simulink subsystem "HeaterDummy"  (R2024b)
settings: Solver=VariableStepAuto  StartTime=0.0  StopTime=10.0  RelTol=1e-3
undefined symbols (not defined in the file or in its folder): batteryHeater
libraries: fl_lib x3, nesl_utility x1
Description:
  | Minimal heater stub with fixed electrical load. Draws constant current (P_max/V_nom) when heater is active (cmdHeater=1). Coolant passes through with no heat exchange. Same port interface as Heater.slx.
settings Model: Creator=jjha  LastModifiedBy=jjha

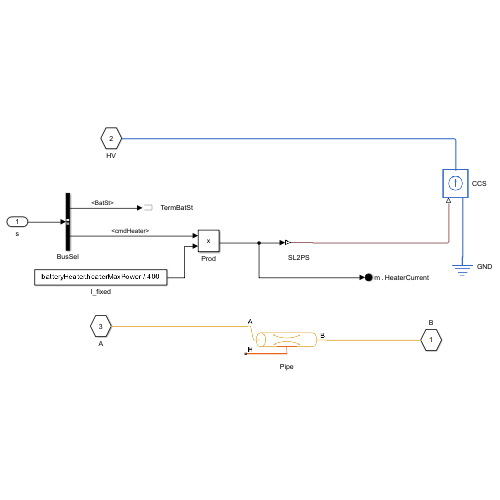
[thumbnail: Simulink's stored preview of the top-level diagram]
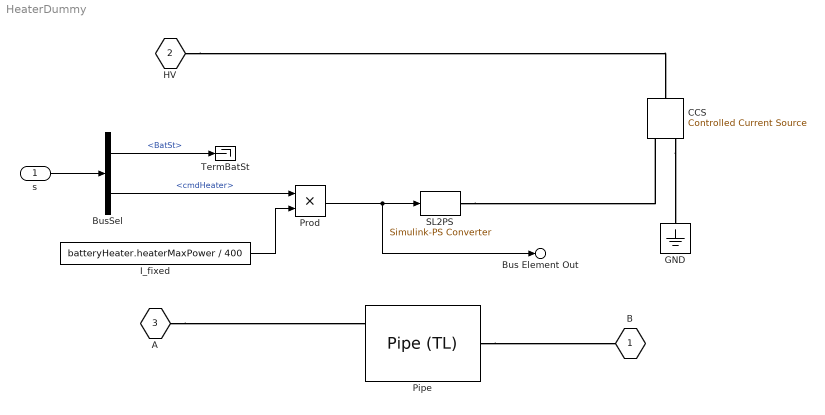
== system HeaterDummy ==
  s : Inport
  BusSel : BusSelector  OutputSignals=BatSt,cmdHeater
  CCS : fl_lib/Electrical/Electrical Sources/Controlled Current Source
  GND : fl_lib/Electrical/Electrical Elements/Electrical Reference
  I_fixed : Constant  Value=batteryHeater.heaterMaxPower / 400
  Pipe : fl_lib/Thermal Liquid/Elements/Pipe (TL)  length=5 m  area=0.01 m^2  Dh=0.1128 m  length_add=1 m  roughness=15e-6 m  Re_lam=2000  Re_tur=4000  shape_factor=64  Nu_lam=3.66  dynamic_compressibility=true  inertia=false  p0=0.101325 MPa  T0=293.15 K  mdot0=0 kg/s
  Prod : Product
  SL2PS : nesl_utility/Simulink-PS Converter  PhysicalDomain=network_engine_domain  SubClassName=ps_input  LeftPortType=input  RightPortType=output  PseudoPeriodic=off  Frequencies=[]  NoiseDistribution=none  NoiseParameters=[]  Unit=1  AffineConversion=off  FilteringAndDerivatives=provide  SimscapeFilterOrder=1  InputFilterTimeConstant=0.001  UdotUserProvided=0
  TermBatSt : Terminator
  B : PMIOPort  Side=Right
  HV : PMIOPort  Port=2  Side=Right
  A : PMIOPort  Port=3  Side=Right
  Bus Element Out : Outport  PortName=m  Element=HeaterCurrent
  wires:
  s/1 -> BusSel/1
  BusSel/1 -> TermBatSt/1  "<BatSt>"
  BusSel/2 -> Prod/1  "<cmdHeater>"
  I_fixed/1 -> Prod/2
  Prod/1 -> SL2PS/1, Bus Element Out/1
  connections:
  CCS/RConn2 -- GND/LConn1
  HV/RConn1 -- CCS/LConn1
  SL2PS/RConn1 -- CCS/RConn1
  A/RConn1 -- Pipe/LConn1
  Pipe/RConn1 -- B/RConn1
